simulink model "fig2_21_simulink"  (R2021b)
settings: Solver=ode45  StartTime=0.0  StopTime=100  RelTol=1e-3  EnableMultiTasking=on
values from neighbouring files (symbols this model uses):
  r = 0.5    [fig2_22.m]    (also in fig2_23.m = 30; fig2_24.m = 30)
settings Model: Creator=One Informatic  LastModifiedBy=One Informatic
settings DataIOCC: LimitDataPoints=on  SaveFormat=Array  SignalLoggingSaveFormat=ModelDataLogs  ReturnWorkspaceOutputs=off  SignalLoggingName=sigsOut
settings DebuggingCC: SaveWithParameterizedLinksMsg=none  UnderspecifiedInitializationDetection=Classic  MergeDetectMultiDrivingBlocksExec=none  SignalResolutionControl=TryResolveAllWithWarning  MultiTaskDSMMsg=warning  MultiTaskCondExecSysMsg=none
settings HardwareCC: ProdBitPerPointer=32  ProdBitPerSizeT=32  ProdBitPerPtrDiffT=32  ProdLargestAtomicFloat=None  ProdIntDivRoundTo=Undefined  ProdEndianess=Unspecified  ProdWordSize=32  ProdHWDeviceType=32-bit Generic  TargetUnknown=on
settings ModelReferenceCC: PropagateSignalLabelsOutOfModel=off
settings GRTTargetCC: CombineOutputUpdateFcns=off  GRTInterface=on
settings ConfigComp: CovMetricSettings=dw  CovSaveCumulativeToWorkspaceVar=on  CovSaveSingleToWorkspaceVar=on

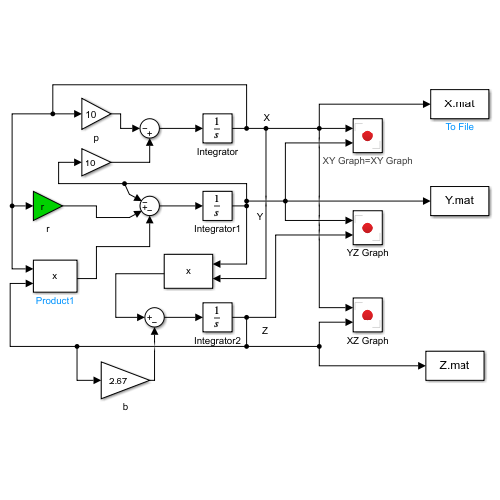
[thumbnail: Simulink's stored preview of the top-level diagram]
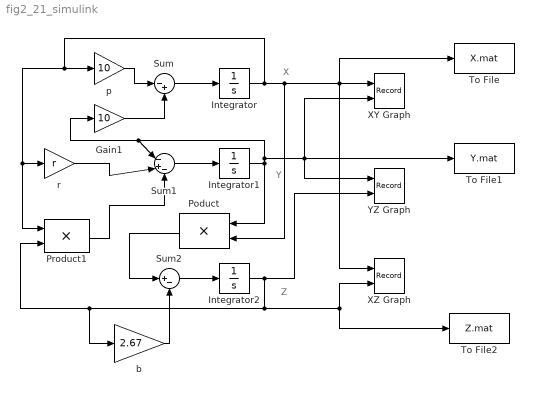
== system fig2_21_simulink ==
  note: X
  note: Y
  note: Z
  Gain1 : Gain  Gain=10  SaturateOnIntegerOverflow=on  OutDataTypeStr=Inherit: Same as input  ParamDataTypeStr=Inherit: Same as input
  Integrator : Integrator  InitialCondition=0.6
  Integrator1 : Integrator  InitialCondition=-10
  Integrator2 : Integrator  InitialCondition=30
  Poduct : Product  SaturateOnIntegerOverflow=on  OutDataTypeStr=Inherit: Same as first input
  Product1 : Product  SaturateOnIntegerOverflow=on  OutDataTypeStr=Inherit: Same as first input
  Sum : Sum  Inputs=|-+  SaturateOnIntegerOverflow=on
  Sum1 : Sum  Inputs=|-+-  SaturateOnIntegerOverflow=on
  Sum2 : Sum  Inputs=|+-  SaturateOnIntegerOverflow=on
  To File : ToFile  Filename=X.mat  MatrixName=X  SampleTime=0.001
  To File1 : ToFile  Filename=Y.mat  MatrixName=Y  SampleTime=0.001
  To File2 : ToFile  Filename=Z.mat  MatrixName=Z  SampleTime=0.001
  XY Graph : Record  FileSettingsInternal="{\"entries\":[{\"content\":{\"excelSettings\":{\"content\":{},\"type\":\"Streamout.ExcelSettings\"}},\"type\":\"Streamout.FileSettingStorage\",\"uuid\":\"7c209d20-3f2c-4cda-9f27-f443970fdfbd\"}],\"packageUris\":[\"http://schema.mathworks.com/mf0/streamout_blocks/R2020a\"],\"version\":\"1.0\"}"  Layout=[1 1]  SignalsInternal="{\"entries\":[{\"content\":{\"signals\":[{\"content\":{\"blockPath\":[\"fig2_21_simulink/XY Graph\"],\"channel\":[],\"dimensions\":[1],\"domain\":\"fig2_21_simulink/XY Graph\",\"lineColor\":\"#a2142f\",\"plots\":[1],\"port\":1,\"sid\":[\"\"],\"signalID\":3700,\"signalName\":\"Integrator\"},\"type\":\"RecordBlkView.Signal\",\"uuid\":\"48b04296-ba91-45b8-aaa5-ebea06843d4c\"},{\"content\":{\"blockPath\":[\"fig2_21_simulink/XY Graph\"],\"channel\":[],\"dimensions\":[1],\"domain\":\"fig2_21_simulink/XY Graph\",\"lineColor\":\"#139fff\",\"plots\":[1],\"port\":2,\"sid\":[\"\"],\"signalID\":3704,\"signalName\":\"Integrator1\"},\"type\":\"RecordBlkView.Signal\",\"uuid\":\"0328044f-2313-42b9-a3b5-5732b44643d7\"}]},\"type\":\"RecordBlkView.InputSignals\",\"uuid\":\"61bb8e54-e9e0-4f9c-8851-82a1fb87f8d3\"}],\"packageUris\":[\"http://schema.mathworks.com/mf0/streamout_blocks/R2020a\"],\"version\":\"1.0\"}"  VisualizationBindings="{\"xyplotplugin\":{\"info\":[{\"series\":[{\"bindingParametersList\":[{\"parameter\":\"X-Axis\",\"signalID\":3700,\"signalName\":\"Integrator\"},{\"parameter\":\"Y-Axis\",\"signalID\":3704,\"signalName\":\"Integrator1\"}],\"seriesID\":42464}],\"subplotID\":1}]}}"  CompatibilityTag=XY  st=0.02
      settings: AttributesFormatString=XY Graph=%<Name>
  XZ Graph : Record  FileSettingsInternal="{\"entries\":[{\"content\":{\"excelSettings\":{\"content\":{},\"type\":\"Streamout.ExcelSettings\"}},\"type\":\"Streamout.FileSettingStorage\",\"uuid\":\"ca91021e-d493-4428-a1f3-1e44a7a500ba\"}],\"packageUris\":[\"http://schema.mathworks.com/mf0/streamout_blocks/R2020a\"],\"version\":\"1.0\"}"  Layout=[1 1]  SignalsInternal="{\"entries\":[{\"content\":{\"signals\":[{\"content\":{\"blockPath\":[\"fig2_21_simulink/XZ Graph\"],\"channel\":[],\"dimensions\":[1],\"domain\":\"fig2_21_simulink/XZ Graph\",\"lineColor\":\"#77ac30\",\"plots\":[],\"port\":1,\"sid\":[\"\"],\"signalID\":3708,\"signalName\":\"Integrator\"},\"type\":\"RecordBlkView.Signal\",\"uuid\":\"d938d2da-4cd6-4133-8153-b59006252a33\"},{\"content\":{\"blockPath\":[\"fig2_21_simulink/XZ Graph\"],\"channel\":[],\"dimensions\":[1],\"domain\":\"fig2_21_simulink/XZ Graph\",\"lineColor\":\"#4dbeee\",\"plots\":[],\"port\":2,\"sid\":[\"\"],\"signalID\":3712,\"signalName\":\"Integrator2\"},\"type\":\"RecordBlkView.Signal\",\"uuid\":\"590284a3-25ea-4727-bac0-fe6103235fbe\"}]},\"type\":\"RecordBlkView.InputSignals\",\"uuid\":\"34f2c5d8-1c3e-44e9-9a00-1e54e6f08583\"}],\"packageUris\":[\"http://schema.mathworks.com/mf0/streamout_blocks/R2020a\"],\"version\":\"1.0\"}"  VisualizationBindings="{\"xyplotplugin\":{\"info\":[{\"series\":[],\"subplotID\":1}]}}"  CompatibilityTag=XY  st=0.02
  YZ Graph : Record  FileSettingsInternal="{\"entries\":[{\"content\":{\"excelSettings\":{\"content\":{},\"type\":\"Streamout.ExcelSettings\"}},\"type\":\"Streamout.FileSettingStorage\",\"uuid\":\"1397175e-e139-404e-9e5d-4c49f85c9d54\"}],\"packageUris\":[\"http://schema.mathworks.com/mf0/streamout_blocks/R2020a\"],\"version\":\"1.0\"}"  Layout=[1 1]  SignalsInternal="{\"entries\":[{\"content\":{\"signals\":[{\"content\":{\"blockPath\":[\"fig2_21_simulink/YZ Graph\"],\"channel\":[],\"dimensions\":[1],\"domain\":\"fig2_21_simulink/YZ Graph\",\"lineColor\":\"#a2142f\",\"plots\":[],\"port\":1,\"sid\":[\"\"],\"signalID\":3716,\"signalName\":\"Integrator1\"},\"type\":\"RecordBlkView.Signal\",\"uuid\":\"9d555d33-22ba-464a-b13f-03cacc9bfa88\"},{\"content\":{\"blockPath\":[\"fig2_21_simulink/YZ Graph\"],\"channel\":[],\"dimensions\":[1],\"domain\":\"fig2_21_simulink/YZ Graph\",\"lineColor\":\"#139fff\",\"plots\":[],\"port\":2,\"sid\":[\"\"],\"signalID\":3720,\"signalName\":\"Integrator2\"},\"type\":\"RecordBlkView.Signal\",\"uuid\":\"941ea537-e97b-4063-aaad-5651b1295e44\"}]},\"type\":\"RecordBlkView.InputSignals\",\"uuid\":\"4edb2642-613f-43af-ae9e-b62479539fb4\"}],\"packageUris\":[\"http://schema.mathworks.com/mf0/streamout_blocks/R2020a\"],\"version\":\"1.0\"}"  VisualizationBindings="{\"xyplotplugin\":{\"info\":[{\"series\":[],\"subplotID\":1}]}}"  CompatibilityTag=XY  st=0.02
  b : Gain  Gain=2.67  SaturateOnIntegerOverflow=on  OutDataTypeStr=Inherit: Same as input  ParamDataTypeStr=Inherit: Same as input
  p : Gain  Gain=10  SaturateOnIntegerOverflow=on  OutDataTypeStr=Inherit: Same as input  ParamDataTypeStr=Inherit: Same as input
  r : Gain  Gain=r  SaturateOnIntegerOverflow=on  OutDataTypeStr=Inherit: Same as input  ParamDataTypeStr=Inherit: Same as input
  wires:
  Sum2/1 -> Integrator2/1
  Sum1/1 -> Integrator1/1
  Sum/1 -> Integrator/1
  Integrator/1 -> p/1, r/1, Product1/1, Poduct/2, To File/1, XY Graph/1, XZ Graph/1
  p/1 -> Sum/1
  Gain1/1 -> Sum/2
  Integrator1/1 -> Gain1/1, Sum1/1, XY Graph/2, To File1/1, YZ Graph/1, Poduct/1
  r/1 -> Sum1/2
  Product1/1 -> Sum1/3
  Integrator2/1 -> YZ Graph/2, Product1/2, b/1, To File2/1, XZ Graph/2
  b/1 -> Sum2/2
  Poduct/1 -> Sum2/1
